simulink library "mahoneyAHRSlibrary"  (R2014a)
settings: Solver=ode45  StartTime=0.0  StopTime=10.0  RelTol=1e-3
values from neighbouring files (symbols this model uses):
  controlDT = 1 / 500    (= 0.002)    [setup.m]
undefined symbols (not defined in the file or in its folder): DiscIntNeverNeededParam
libraries: aerolibutil x8, simulink x3, mahoneyAHRSlibrary x1, aerolibtransform2 x1
settings Model: Creator=e722209  LastModifiedBy=John Ihlein

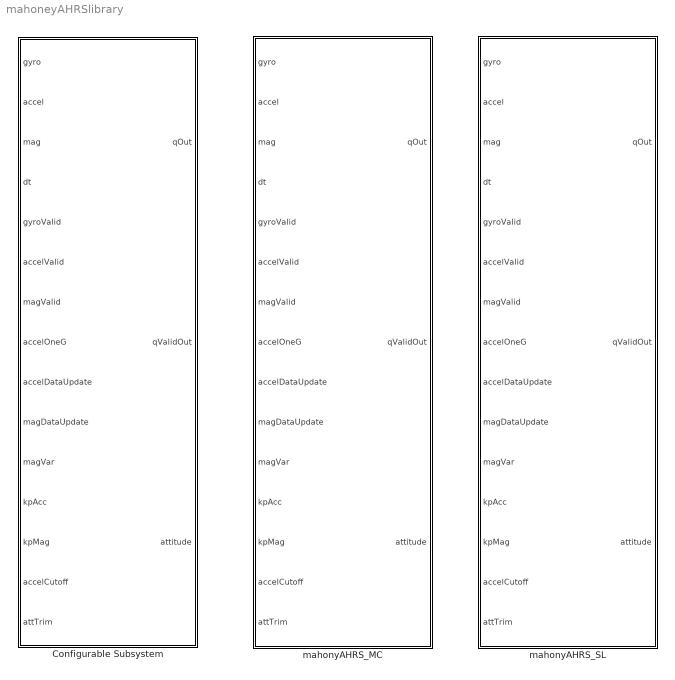
== system mahoneyAHRSlibrary ==
  Configurable Subsystem : Subsystem  BlockChoice=mahonyAHRS_MC
      settings: TemplateBlock=self  MemberBlocks=mahonyAHRS_MC,mahonyAHRS_SL
  mahonyAHRS_MC : MATLAB Function  TreatAsAtomicUnit=on
  mahonyAHRS_SL : Subsystem  TreatAsAtomicUnit=on

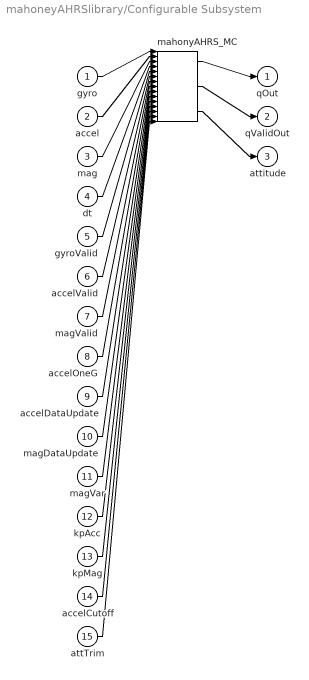
== system mahoneyAHRSlibrary/Configurable Subsystem ==
  gyro : Inport
  accel : Inport  Port=2
  mag : Inport  Port=3
  dt : Inport  Port=4
  gyroValid : Inport  Port=5
  accelValid : Inport  Port=6
  magValid : Inport  Port=7
  accelOneG : Inport  Port=8
  accelDataUpdate : Inport  Port=9
  magDataUpdate : Inport  Port=10
  magVar : Inport  Port=11
  kpAcc : Inport  Port=12
  kpMag : Inport  Port=13
  accelCutoff : Inport  Port=14
  attTrim : Inport  Port=15
  mahonyAHRS_MC : mahoneyAHRSlibrary/mahonyAHRS_MC
  qOut : Outport
  qValidOut : Outport  Port=2
  attitude : Outport  Port=3
  wires:
  gyro/1 -> mahonyAHRS_MC/1
  accel/1 -> mahonyAHRS_MC/2
  mag/1 -> mahonyAHRS_MC/3
  dt/1 -> mahonyAHRS_MC/4
  gyroValid/1 -> mahonyAHRS_MC/5
  accelValid/1 -> mahonyAHRS_MC/6
  magValid/1 -> mahonyAHRS_MC/7
  accelOneG/1 -> mahonyAHRS_MC/8
  accelDataUpdate/1 -> mahonyAHRS_MC/9
  magDataUpdate/1 -> mahonyAHRS_MC/10
  magVar/1 -> mahonyAHRS_MC/11
  kpAcc/1 -> mahonyAHRS_MC/12
  kpMag/1 -> mahonyAHRS_MC/13
  accelCutoff/1 -> mahonyAHRS_MC/14
  attTrim/1 -> mahonyAHRS_MC/15
  mahonyAHRS_MC/1 -> qOut/1
  mahonyAHRS_MC/2 -> qValidOut/1
  mahonyAHRS_MC/3 -> attitude/1

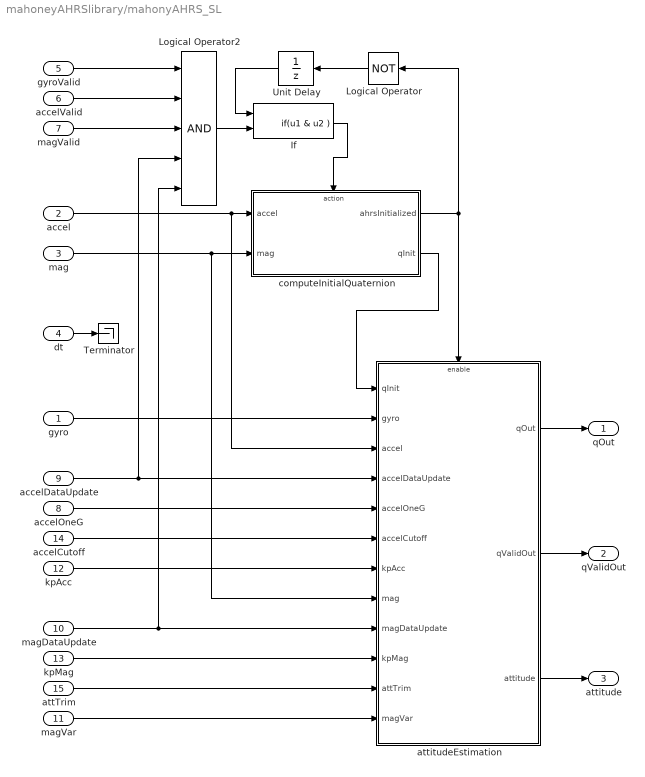
== system mahoneyAHRSlibrary/mahonyAHRS_SL ==
  gyro : Inport
  accel : Inport  Port=2
  mag : Inport  Port=3
  dt : Inport  Port=4
  gyroValid : Inport  Port=5
  accelValid : Inport  Port=6
  magValid : Inport  Port=7
  accelOneG : Inport  Port=8
  accelDataUpdate : Inport  Port=9
  magDataUpdate : Inport  Port=10
  magVar : Inport  Port=11
  kpAcc : Inport  Port=12
  kpMag : Inport  Port=13
  accelCutoff : Inport  Port=14
  attTrim : Inport  Port=15
  If : If  NumInputs=2  IfExpression=u1 & u2  ShowElse=off
  Logical Operator : Logic  Operator=NOT  IconShape=distinctive  AllPortsSameDT=off  OutDataTypeStr=boolean
  Logical Operator2 : Logic  Inputs=5  IconShape=distinctive  AllPortsSameDT=off  OutDataTypeStr=boolean
  Terminator : Terminator
  Unit Delay : UnitDelay  InitialCondition=1  SampleTime=-1
  attitudeEstimation : Subsystem  TreatAsAtomicUnit=on
  computeInitialQuaternion : Subsystem  TreatAsAtomicUnit=on
  qOut : Outport
  qValidOut : Outport  Port=2
  attitude : Outport  Port=3
  wires:
  magVar/1 -> attitudeEstimation/12(magVar)
  attTrim/1 -> attitudeEstimation/11(attTrim)
  attitudeEstimation/2(qValidOut) -> qValidOut/1
  attitudeEstimation/1(qOut) -> qOut/1
  Logical Operator/1 -> Unit Delay/1
  Logical Operator2/1 -> If/2
  computeInitialQuaternion/2(qInit) -> attitudeEstimation/1(qInit)
  Unit Delay/1 -> If/1
  computeInitialQuaternion/1(ahrsInitialized) -> Logical Operator/1, attitudeEstimation/Enable
  If/1 -> computeInitialQuaternion/Action
  attitudeEstimation/3(attitude) -> attitude/1
  accelDataUpdate/1 -> attitudeEstimation/4(accelDataUpdate), Logical Operator2/4
  magDataUpdate/1 -> attitudeEstimation/9(magDataUpdate), Logical Operator2/5
  accelOneG/1 -> attitudeEstimation/5(accelOneG)
  accelCutoff/1 -> attitudeEstimation/6(accelCutoff)
  accel/1 -> attitudeEstimation/3(accel), computeInitialQuaternion/1(accel)
  mag/1 -> attitudeEstimation/8(mag), computeInitialQuaternion/2(mag)
  gyro/1 -> attitudeEstimation/2(gyro)
  gyroValid/1 -> Logical Operator2/1
  magValid/1 -> Logical Operator2/3
  accelValid/1 -> Logical Operator2/2
  kpMag/1 -> attitudeEstimation/10(kpMag)
  kpAcc/1 -> attitudeEstimation/7(kpAcc)
  dt/1 -> Terminator/1

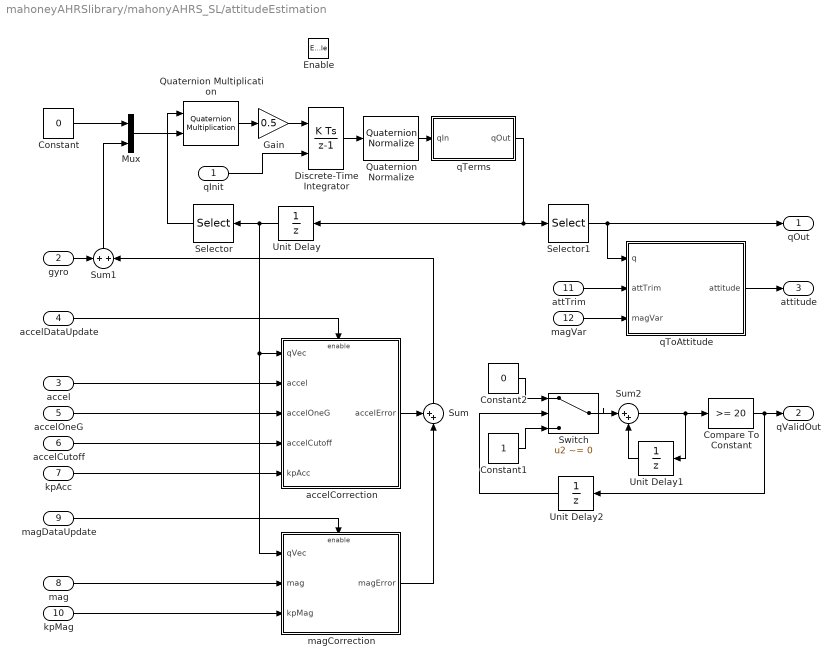
== system mahoneyAHRSlibrary/mahonyAHRS_SL/attitudeEstimation ==
  qInit : Inport
  gyro : Inport  Port=2
  accel : Inport  Port=3
  accelDataUpdate : Inport  Port=4
  accelOneG : Inport  Port=5
  accelCutoff : Inport  Port=6
  kpAcc : Inport  Port=7
  mag : Inport  Port=8
  magDataUpdate : Inport  Port=9
  kpMag : Inport  Port=10
  attTrim : Inport  Port=11
  magVar : Inport  Port=12
  Enable : EnablePort
  Compare To Constant : simulink/Logic and Bit Operations/Compare To Constant  relop=>=  const=20  OutDataTypeStr=uint8
  Constant : Constant  Value=0  OutDataTypeStr=single  SampleTime=controlDT
  Constant1 : Constant  OutDataTypeStr=single  SampleTime=controlDT
  Constant2 : Constant  Value=0  OutDataTypeStr=single  SampleTime=controlDT
  Discrete-Time Integrator : DiscreteIntegrator  InitialConditionSource=external  SampleTime=controlDT  ICPrevOutput=DiscIntNeverNeededParam  ICPrevScaledInput=DiscIntNeverNeededParam
  Gain : Gain  Gain=0.5
  Mux : Mux  Inputs=[1 3]
  Quaternion Multiplication : aerolibutil/Quaternion Multiplication
  Quaternion Normalize : aerolibutil/Quaternion Normalize
  Selector : Selector  InputPortWidth=14  Indices=[1:4]
  Selector1 : Selector  InputPortWidth=14  Indices=[1:4]
  Sum : Sum  Inputs=++|
  Sum1 : Sum  Inputs=+|+
  Sum2 : Sum  Inputs=|++
  Switch : Switch  Criteria=u2 ~= 0
  Unit Delay : UnitDelay  InitialCondition=[1 0 0 0 1 0 0 0 0 0 0 0 0 0]  SampleTime=-1
  Unit Delay1 : UnitDelay  SampleTime=-1
  Unit Delay2 : UnitDelay  SampleTime=-1
  accelCorrection : Subsystem  TreatAsAtomicUnit=on
  magCorrection : Subsystem  TreatAsAtomicUnit=on
  qTerms : Subsystem
  qToAttitude : Subsystem
  qOut : Outport  InitialOutput=[1 0 0 0]
  qValidOut : Outport  Port=2
  attitude : Outport  Port=3
  wires:
  magVar/1 -> qToAttitude/3(magVar)
  attTrim/1 -> qToAttitude/2(attTrim)
  qToAttitude/1(attitude) -> attitude/1
  Unit Delay2/1 -> Switch/2
  Compare To Constant/1 -> Unit Delay2/1, qValidOut/1
  Sum2/1 -> Unit Delay1/1, Compare To Constant/1
  Constant2/1 -> Switch/1
  Constant1/1 -> Switch/3
  Switch/1 -> Sum2/1
  Unit Delay1/1 -> Sum2/2
  Constant/1 -> Mux/1
  Mux/1 -> Quaternion Multiplication/2
  Unit Delay/1 -> accelCorrection/1(qVec), magCorrection/1(qVec), Selector/1
  Selector/1 -> Quaternion Multiplication/1
  Discrete-Time Integrator/1 -> Quaternion Normalize/1
  Selector1/1 -> qOut/1, qToAttitude/1(q)
  Quaternion Normalize/1 -> qTerms/1(qIn)
  qTerms/1(qOut) -> Selector1/1, Unit Delay/1
  qInit/1 -> Discrete-Time Integrator/2
  mag/1 -> magCorrection/2(mag)
  accel/1 -> accelCorrection/2(accel)
  accelOneG/1 -> accelCorrection/3(accelOneG)
  accelCutoff/1 -> accelCorrection/4(accelCutoff)
  Quaternion Multiplication/1 -> Gain/1
  Gain/1 -> Discrete-Time Integrator/1
  gyro/1 -> Sum1/1
  Sum1/1 -> Mux/2
  Sum/1 -> Sum1/2
  accelCorrection/1(accelError) -> Sum/1
  accelDataUpdate/1 -> accelCorrection/Enable
  magCorrection/1(magError) -> Sum/2
  magDataUpdate/1 -> magCorrection/Enable
  kpAcc/1 -> accelCorrection/5(kpAcc)
  kpMag/1 -> magCorrection/3(kpMag)

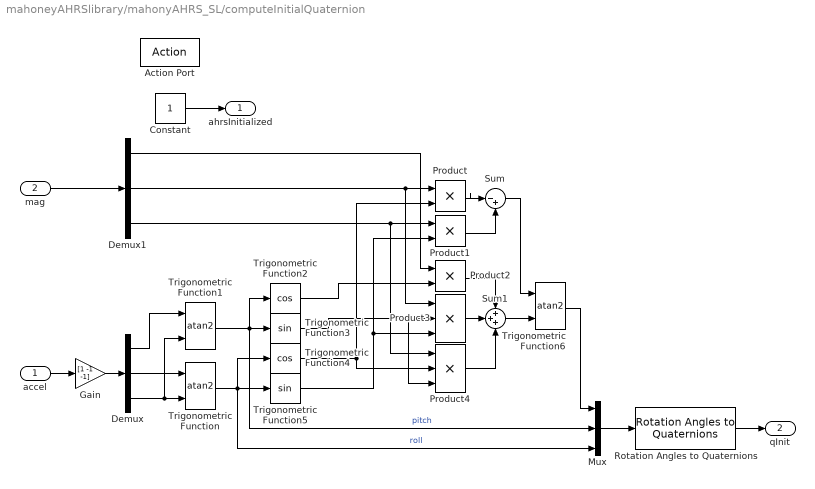
== system mahoneyAHRSlibrary/mahonyAHRS_SL/computeInitialQuaternion ==
  accel : Inport
  mag : Inport  Port=2
  Action Port : ActionPort
  Constant : Constant  OutDataTypeStr=uint8
  Demux : Demux  Outputs=3
  Demux1 : Demux  Outputs=3
  Gain : Gain  Gain=[1 -1 -1]
  Mux : Mux  Inputs=3
  Product : Product
  Product1 : Product
  Product2 : Product
  Product3 : Product  Inputs=3
  Product4 : Product  Inputs=3
  Rotation Angles to Quaternions : aerolibtransform2/Rotation Angles to Quaternions  rotationOrder=ZYX
  Sum : Sum  Inputs=|-+
  Sum1 : Sum  Inputs=+++
  Trigonometric Function : Trigonometry  Operator=atan2
  Trigonometric Function1 : Trigonometry  Operator=atan2
  Trigonometric Function2 : Trigonometry  Operator=cos
  Trigonometric Function3 : Trigonometry
  Trigonometric Function4 : Trigonometry  Operator=cos
  Trigonometric Function5 : Trigonometry
  Trigonometric Function6 : Trigonometry  Operator=atan2
  ahrsInitialized : Outport  InitialOutput=0
  qInit : Outport  Port=2  InitialOutput=[1 0 0 0]
  wires:
  Constant/1 -> ahrsInitialized/1
  accel/1 -> Gain/1
  Gain/1 -> Demux/1
  Demux/3 -> Trigonometric Function1/2, Trigonometric Function/2
  Demux/2 -> Trigonometric Function/1
  Demux/1 -> Trigonometric Function1/1
  Trigonometric Function/1 -> Mux/3, Trigonometric Function4/1, Trigonometric Function5/1  "roll"
  Trigonometric Function1/1 -> Trigonometric Function2/1, Mux/2, Trigonometric Function3/1  "pitch"
  mag/1 -> Demux1/1
  Demux1/2 -> Product3/1, Product/1
  Trigonometric Function4/1 -> Product4/2, Product/2
  Demux1/3 -> Product4/1, Product1/1
  Trigonometric Function5/1 -> Product3/3, Product1/2
  Product/1 -> Sum/1
  Product1/1 -> Sum/2
  Demux1/1 -> Product2/1
  Trigonometric Function2/1 -> Product2/2
  Trigonometric Function3/1 -> Product4/3, Product3/2
  Product3/1 -> Sum1/2
  Product2/1 -> Sum1/1
  Product4/1 -> Sum1/3
  Sum1/1 -> Trigonometric Function6/2
  Sum/1 -> Trigonometric Function6/1
  Mux/1 -> Rotation Angles to Quaternions/1
  Trigonometric Function6/1 -> Mux/1
  Rotation Angles to Quaternions/1 -> qInit/1

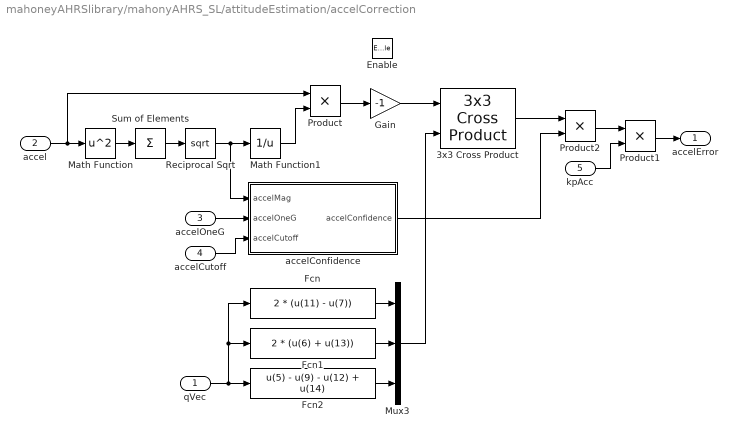
== system mahoneyAHRSlibrary/mahonyAHRS_SL/attitudeEstimation/accelCorrection ==
  qVec : Inport
  accel : Inport  Port=2
  accelOneG : Inport  Port=3
  accelCutoff : Inport  Port=4
  kpAcc : Inport  Port=5
  Enable : EnablePort
  3x3 Cross Product : aerolibutil/3x3 Cross Product
  Fcn : Fcn  Expr=2 * (u(11) - u(7))
  Fcn1 : Fcn  Expr=2 * (u(6) + u(13))
  Fcn2 : Fcn  Expr=u(5) - u(9) - u(12) + u(14)
  Gain : Gain  Gain=-1
  Math Function : Math  Operator=square  SaturateOnIntegerOverflow=on
  Math Function1 : Math  Operator=reciprocal  SaturateOnIntegerOverflow=on
  Mux3 : Mux  Inputs=3
  Product : Product
  Product1 : Product
  Product2 : Product
  Reciprocal Sqrt : Sqrt  SaturateOnIntegerOverflow=on
  Sum of Elements : Sum  Inputs=+
  accelConfidence : Subsystem
  accelError : Outport
  wires:
  accel/1 -> Product/1, Math Function/1
  Math Function/1 -> Sum of Elements/1
  Sum of Elements/1 -> Reciprocal Sqrt/1
  Reciprocal Sqrt/1 -> accelConfidence/1(accelMag), Math Function1/1
  Math Function1/1 -> Product/2
  accelOneG/1 -> accelConfidence/2(accelOneG)
  accelCutoff/1 -> accelConfidence/3(accelCutoff)
  Fcn/1 -> Mux3/1
  Fcn1/1 -> Mux3/2
  Fcn2/1 -> Mux3/3
  qVec/1 -> Fcn1/1, Fcn/1, Fcn2/1
  Product/1 -> Gain/1
  Gain/1 -> 3x3 Cross Product/1
  Mux3/1 -> 3x3 Cross Product/2
  Product2/1 -> Product1/1
  kpAcc/1 -> Product1/2
  Product1/1 -> accelError/1
  accelConfidence/1(accelConfidence) -> Product2/2
  3x3 Cross Product/1 -> Product2/1

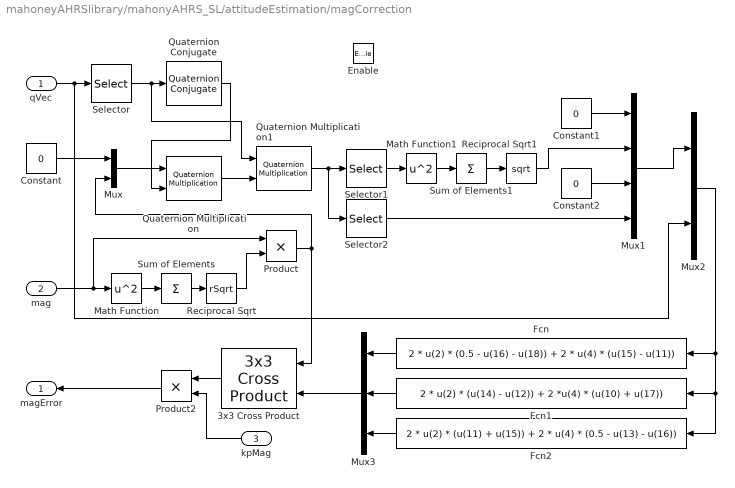
== system mahoneyAHRSlibrary/mahonyAHRS_SL/attitudeEstimation/magCorrection ==
  qVec : Inport
  mag : Inport  Port=2
  kpMag : Inport  Port=3
  Enable : EnablePort
  3x3 Cross Product : aerolibutil/3x3 Cross Product
  Constant : Constant  Value=0  OutDataTypeStr=single  SampleTime=controlDT
  Constant1 : Constant  Value=0  OutDataTypeStr=single  SampleTime=controlDT
  Constant2 : Constant  Value=0  OutDataTypeStr=single  SampleTime=controlDT
  Fcn : Fcn  Expr=2 * u(2) * (0.5 - u(16) - u(18)) + 2 * u(4) * (u(15) - u(11))
  Fcn1 : Fcn  Expr=2 * u(2) * (u(14) - u(12)) + 2 *u(4) * (u(10) + u(17))
  Fcn2 : Fcn  Expr=2 * u(2) * (u(11) + u(15)) + 2 * u(4) * (0.5 - u(13) - u(16))
  Math Function : Math  Operator=square  SaturateOnIntegerOverflow=on
  Math Function1 : Math  Operator=square  SaturateOnIntegerOverflow=on
  Mux : Mux  Inputs=[1 3]
  Mux1 : Mux
  Mux2 : Mux  Inputs=2
  Mux3 : Mux  Inputs=3
  Product : Product
  Product2 : Product
  Quaternion Conjugate : aerolibutil/Quaternion Conjugate
  Quaternion Multiplication : aerolibutil/Quaternion Multiplication
  Quaternion Multiplication1 : aerolibutil/Quaternion Multiplication
  Reciprocal Sqrt : Sqrt  Operator=rSqrt  SaturateOnIntegerOverflow=on
  Reciprocal Sqrt1 : Sqrt  SaturateOnIntegerOverflow=on
  Selector : Selector  InputPortWidth=14  Indices=[1:4]
  Selector1 : Selector  InputPortWidth=4  Indices=[2 3]
  Selector2 : Selector  InputPortWidth=4  Indices=4
  Sum of Elements : Sum  Inputs=+
  Sum of Elements1 : Sum  Inputs=+
  magError : Outport
  wires:
  qVec/1 -> Mux2/2, Selector/1
  mag/1 -> Product/1, Math Function/1
  Math Function/1 -> Sum of Elements/1
  Sum of Elements/1 -> Reciprocal Sqrt/1
  Reciprocal Sqrt/1 -> Product/2
  Constant/1 -> Mux/1
  Mux/1 -> Quaternion Multiplication/1
  Selector/1 -> Quaternion Multiplication1/1, Quaternion Conjugate/1
  Quaternion Conjugate/1 -> Quaternion Multiplication/2
  Quaternion Multiplication/1 -> Quaternion Multiplication1/2
  Selector1/1 -> Math Function1/1
  Math Function1/1 -> Sum of Elements1/1
  Sum of Elements1/1 -> Reciprocal Sqrt1/1
  Product/1 -> Mux/2, 3x3 Cross Product/1
  Quaternion Multiplication1/1 -> Selector2/1, Selector1/1
  Reciprocal Sqrt1/1 -> Mux1/2
  Constant2/1 -> Mux1/3
  Constant1/1 -> Mux1/1
  Selector2/1 -> Mux1/4
  Mux1/1 -> Mux2/1
  Mux2/1 -> Fcn2/1, Fcn1/1, Fcn/1
  Fcn/1 -> Mux3/1
  Fcn1/1 -> Mux3/2
  Fcn2/1 -> Mux3/3
  3x3 Cross Product/1 -> Product2/1
  Product2/1 -> magError/1
  Mux3/1 -> 3x3 Cross Product/2
  kpMag/1 -> Product2/2

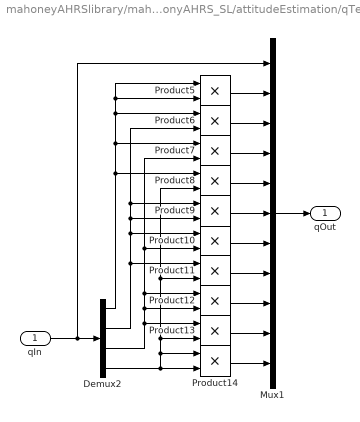
== system mahoneyAHRSlibrary/mahonyAHRS_SL/attitudeEstimation/qTerms ==
  qIn : Inport
  Demux2 : Demux
  Mux1 : Mux  Inputs=[4 1 1 1 1 1 1 1 1 1 1]
  Product{5..14} (10 alike) : Product
  qOut : Outport
  wires:
  Demux2/3 -> Product13/1, Product12/2, Product12/1, Product10/2, Product7/2
  Product7/1 -> Mux1/4
  Product10/1 -> Mux1/7
  Mux1/1 -> qOut/1
  Product11/1 -> Mux1/8
  Product6/1 -> Mux1/3
  Product5/1 -> Mux1/2
  Demux2/4 -> Product14/2, Product14/1, Product13/2, Product11/2, Product8/2
  Product14/1 -> Mux1/11
  Product12/1 -> Mux1/9
  qIn/1 -> Demux2/1, Mux1/1
  Product13/1 -> Mux1/10
  Product8/1 -> Mux1/5
  Product9/1 -> Mux1/6
  Demux2/1 -> Product8/1, Product7/1, Product6/1, Product5/2, Product5/1
  Demux2/2 -> Product11/1, Product10/1, Product9/2, Product9/1, Product6/2

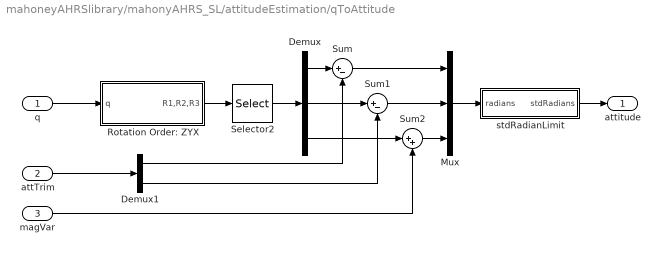
== system mahoneyAHRSlibrary/mahonyAHRS_SL/attitudeEstimation/qToAttitude ==
  q : Inport
  attTrim : Inport  Port=2
  magVar : Inport  Port=3
  Demux : Demux  Outputs=3
  Demux1 : Demux  Outputs=2
  Mux : Mux  Inputs=3
  Rotation Order: ZYX : Subsystem
  Selector2 : Selector  InputPortWidth=3  Indices=[3 2 1]
  Sum : Sum  Inputs=|+-
  Sum1 : Sum  Inputs=|+-
  Sum2 : Sum  Inputs=|++
  stdRadianLimit : Subsystem
  attitude : Outport
  wires:
  attTrim/1 -> Demux1/1
  magVar/1 -> Sum2/2
  Demux1/2 -> Sum1/2
  Demux1/1 -> Sum/2
  Demux/3 -> Sum2/1
  Sum1/1 -> Mux/2
  Demux/2 -> Sum1/1
  Demux/1 -> Sum/1
  Sum/1 -> Mux/1
  Sum2/1 -> Mux/3
  Selector2/1 -> Demux/1
  Mux/1 -> stdRadianLimit/1(radians)
  q/1 -> Rotation Order: ZYX/1(q)
  stdRadianLimit/1(stdRadians) -> attitude/1
  Rotation Order: ZYX/1(R1,R2,R3) -> Selector2/1

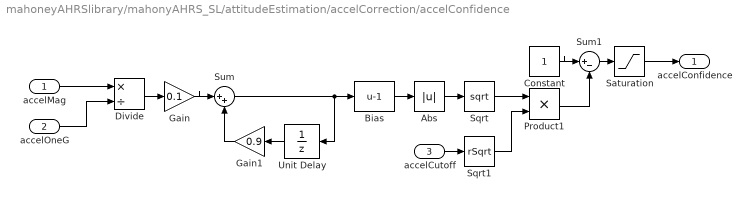
== system mahoneyAHRSlibrary/mahonyAHRS_SL/attitudeEstimation/accelCorrection/accelConfidence ==
  accelMag : Inport
  accelOneG : Inport  Port=2
  accelCutoff : Inport  Port=3
  Abs : Abs
  Bias : Bias  Bias=-1
  Constant : Constant  OutDataTypeStr=single  SampleTime=controlDT
  Divide : Product  Inputs=*/
  Gain : Gain  Gain=0.1
  Gain1 : Gain  Gain=0.9
  Product1 : Product
  Saturation : Saturate  UpperLimit=1  LowerLimit=0
  Sqrt : Sqrt  SaturateOnIntegerOverflow=on
  Sqrt1 : Sqrt  Operator=rSqrt  SaturateOnIntegerOverflow=on
  Sum : Sum  Inputs=|++
  Sum1 : Sum  Inputs=|+-
  Unit Delay : UnitDelay  InitialCondition=1  SampleTime=-1
  accelConfidence : Outport
  wires:
  Gain1/1 -> Sum/2
  Abs/1 -> Sqrt/1
  Gain/1 -> Sum/1
  Divide/1 -> Gain/1
  Bias/1 -> Abs/1
  Unit Delay/1 -> Gain1/1
  Sum/1 -> Bias/1, Unit Delay/1
  Product1/1 -> Sum1/2
  Sqrt/1 -> Product1/1
  accelCutoff/1 -> Sqrt1/1
  Constant/1 -> Sum1/1
  Sum1/1 -> Saturation/1
  accelOneG/1 -> Divide/2
  Saturation/1 -> accelConfidence/1
  accelMag/1 -> Divide/1
  Sqrt1/1 -> Product1/2

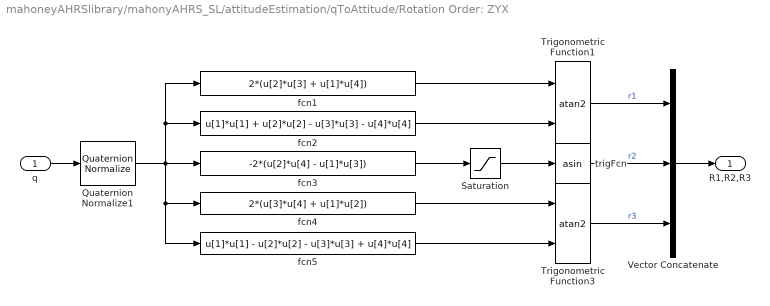
== system mahoneyAHRSlibrary/mahonyAHRS_SL/attitudeEstimation/qToAttitude/Rotation Order: ZYX ==
  q : Inport
  Quaternion Normalize1 : aerolibutil/Quaternion Normalize
  Saturation : Saturate  UpperLimit=1  LowerLimit=-1
  Trigonometric Function1 : Trigonometry  Operator=atan2
  Trigonometric Function3 : Trigonometry  Operator=atan2
  Vector Concatenate : Concatenate  NumInputs=3
  fcn1 : Fcn  Expr=2*(u[2]*u[3] + u[1]*u[4])
  fcn2 : Fcn  Expr=u[1]*u[1] + u[2]*u[2] - u[3]*u[3] - u[4]*u[4]
  fcn3 : Fcn  Expr=-2*(u[2]*u[4] - u[1]*u[3])
  fcn4 : Fcn  Expr=2*(u[3]*u[4] + u[1]*u[2])
  fcn5 : Fcn  Expr=u[1]*u[1] - u[2]*u[2] - u[3]*u[3] + u[4]*u[4]
  trigFcn : Trigonometry  Operator=asin
  R1,R2,R3 : Outport
  wires:
  Quaternion Normalize1/1 -> fcn3/1, fcn4/1, fcn5/1, fcn2/1, fcn1/1
  Trigonometric Function3/1 -> Vector Concatenate/3  "r3"
  trigFcn/1 -> Vector Concatenate/2  "r2"
  Trigonometric Function1/1 -> Vector Concatenate/1  "r1"
  Vector Concatenate/1 -> R1,R2,R3/1
  q/1 -> Quaternion Normalize1/1
  fcn3/1 -> Saturation/1
  fcn1/1 -> Trigonometric Function1/1
  fcn2/1 -> Trigonometric Function1/2
  fcn4/1 -> Trigonometric Function3/1
  fcn5/1 -> Trigonometric Function3/2
  Saturation/1 -> trigFcn/1

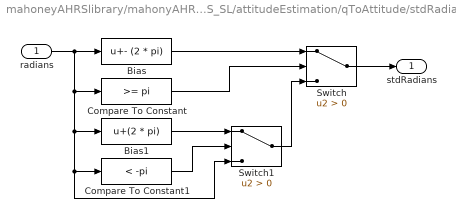
== system mahoneyAHRSlibrary/mahonyAHRS_SL/attitudeEstimation/qToAttitude/stdRadianLimit ==
  radians : Inport
  Bias : Bias  Bias=- (2 * pi)
  Bias1 : Bias  Bias=(2 * pi)
  Compare To Constant : simulink/Logic and Bit Operations/Compare To Constant  relop=>=  const=pi  OutDataTypeStr=boolean
  Compare To Constant1 : simulink/Logic and Bit Operations/Compare To Constant  relop=<  const=-pi  OutDataTypeStr=boolean
  Switch : Switch  Criteria=u2 > Threshold
  Switch1 : Switch  Criteria=u2 > Threshold
  stdRadians : Outport
  wires:
  Switch/1 -> stdRadians/1
  radians/1 -> Bias/1, Compare To Constant/1, Bias1/1, Compare To Constant1/1, Switch1/3
  Switch1/1 -> Switch/3
  Compare To Constant1/1 -> Switch1/2
  Bias1/1 -> Switch1/1
  Bias/1 -> Switch/1
  Compare To Constant/1 -> Switch/2

== matlab function mahoneyAHRSlibrary/mahonyAHRS_MC ==
  data: gyro input; qOut output; accel input; mag input; dt input; gyroValid input; accelValid input; magValid input; accelOneG input; accelDataUpdate input; magDataUpdate input; magVar input; kpAcc input; kpMag input; qValidOut output; accelCutoff input; attitude output; attTrim input
%%%%%%%%%%%%%%%%%%%%%%%%%%%%%%%%%%%%%%%%%%%%%%%%%%%%%%%%%%%%%%%%%%%%%%%
% MAYHONYAHRS Madgwick's implementation of Mayhony's AHRS algorithm
%
%   Date          Author          Notes
%   28/09/2011    SOH Madgwick    Initial release
%   25/08/2014    J Ihlein        Integrated into FF32
%%%%%%%%%%%%%%%%%%%%%%%%%%%%%%%%%%%%%%%%%%%%%%%%%%%%%%%%%%%%%%%%%%%%%%%

function [qOut, qValidOut, attitude] = mahonyAHRS(gyro, accel, mag, dt,...
                                                  gyroValid, accelValid, magValid,...
                                                  accelOneG, accelDataUpdate,...
                                                  magDataUpdate, magVar, ...
                                                  kpAcc, kpMag, accelCutoff, attTrim)
%#codegen

%%%%%%%%%%%%%%%%%%%%%%%%%%%%%%%%%%%%%%%%%%%%%%%%%%%%%%%%%%%

persistent accelConfidenceDecay ahrsFirstPass eAcc eMag pastAccelFilter
persistent q qValid qValidCount
persistent q1q1 q1q2 q1q3 q1q4 
persistent q2q2 q2q3 q2q4
persistent q3q3 q3q4
persistent q4q4

if isempty(ahrsFirstPass)
    accelConfidenceDecay = single(0);
    ahrsFirstPass        = uint8(1);
    eAcc                 = single([0 0 0]');
    eMag                 = single([0 0 0]');
    pastAccelFilter      = single(1);
    q                    = single([1 0 0 0]);
    qValid               = uint8(0);
    qValidCount          = uint8(0);
    
    q1q1 = single(1);
    q1q2 = single(0);
    q1q3 = single(0);
    q1q4 = single(0);
    q2q2 = single(0);
    q2q3 = single(0);
    q2q4 = single(0);
    q3q3 = single(0);
    q3q4 = single(0);
    q4q4 = single(0);
end

%%%%%%%%%%%%%%%%%%%%%%%%%%%%%%%%%%%%%%%%%%%%%%%%%%%%%%%%%%%

attitude = single([0 0 0]);

%%%%%%%%%%%%%%%%%%%%%%%%%%%%%%%%%%%%%%%%%%%%%%%%%%%%%%%%%%%

if ahrsFirstPass && accelValid && accelDataUpdate && gyroValid && magValid && magDataUpdate
    initialRoll  = atan2(-accel(2), -accel(3));
    initialPitch = atan2( accel(1), -accel(3));
    
    cosRoll  = cos(initialRoll);
    sinRoll  = sin(initialRoll);
    cosPitch = cos(initialPitch);
    sinPitch = sin(initialPitch);
    
    magX = mag(1) * cosPitch + mag(2) * sinRoll * sinPitch + mag(3) * cosRoll * sinPitch;
    magY = mag(2) * cosRoll - mag(3) * sinRoll;
    
    initialHdg = atan2(-magY, magX);
    
    u1 = sin(initialHdg   / 2);
    u2 = sin(initialPitch / 2);
    u3 = sin(initialRoll  / 2);
    u4 = cos(initialHdg   / 2);
    u5 = cos(initialPitch / 2);
    u6 = cos(initialRoll  / 2);
    
    q(1) = u4 * u5 * u6 + u1 * u2 * u3;
    q(2) = u4 * u5 * u3 - u1 * u2 * u6;
    q(3) = u4 * u2 * u6 + u1 * u5 * u3;
    q(4) = u1 * u5 * u6 - u4 * u2 * u3;
    
    q1q1 = q(1) * q(1);
    q1q2 = q(1) * q(2);
    q1q3 = q(1) * q(3);
    q1q4 = q(1) * q(4);
    q2q2 = q(2) * q(2);
    q2q3 = q(2) * q(3);
    q2q4 = q(2) * q(4);
    q3q3 = q(3) * q(3);
    q3q4 = q(3) * q(4);
    q4q4 = q(4) * q(4);
    
    accelConfidenceDecay = single(1) / sqrt(accelCutoff);
    
    ahrsFirstPass = uint8(0);
end

%%%%%%%%%%%%%%%%%%%%%%%%%%%%%%%%%%%%%%%%%%%%%%%%%%%%%%%%%%%

if ~ahrsFirstPass
    if accelDataUpdate
        %Normalise accelerometer measurement
        accelNorm = norm(accel);
        % if(accelNorm == 0), return; end   % handle NaN
        accel = accel / accelNorm;          % normalise magnitude
        
        input = accelNorm / accelOneG;
        output = 0.1 * input + 0.9 * pastAccelFilter;
        pastAccelFilter = output;
        accelConfidence = 1 - (accelConfidenceDecay * sqrt(abs(output - 1)));
        
        if accelConfidence > 1
            accelConfidence = single(1);
        elseif accelConfidence < 0
            accelConfidence = single(0);
        end
        
        % Estimated direction of gravity and magnetic field
        v = [2 * (q2q4 - q1q3)
             2 * (q1q2 + q3q4)
             q1q1 - q2q2 - q3q3 + q4q4];
        
        % Error is sum of cross product between estimated direction and measured direction of fields
        eAcc = cross(-accel, v) * kpAcc * accelConfidence;
    end
    
    %%%%%%%%%%%%%%%%%%%%%%%%%%%%%%%%%%%%%%%%%%%%%%%%%%%%%%%
    
    if magDataUpdate
        % Normalise magnetometer measurement
        % if(norm(mag) == 0), return; end     % handle NaN
        mag = mag / norm(mag);                % normalise magnitude
        
        % Reference direction of Earth's magnetic field
        h = quaternProd(q, quaternProd([0 mag'], quaternConj(q)));
        b = [0 norm([h(2) h(3)]) 0 h(4)];
        
        w = [2 * b(2) * (0.5 - q3q3 - q4q4) + 2 * b(4) * (q2q4 - q1q3)
             2 * b(2) * (q2q3 - q1q4) + 2 * b(4) * (q1q2 + q3q4)
             2 * b(2) * (q1q3 + q2q4) + 2 * b(4) * (0.5 - q2q2 - q3q3)];
        
        % Error is sum of cross product between estimated direction and measured direction of fields
        eMag = cross(mag, w) * kpMag;
    end
    
    %%%%%%%%%%%%%%%%%%%%%%%%%%%%%%%%%%%%%%%%%%%%%%%%%%%%%%%
    
    % Apply feedback terms
    gyro = gyro + eAcc + eMag;
    
    % Compute rate of change of quaternion
    qDot = 0.5 * quaternProd(q, [0 gyro(1) gyro(2) gyro(3)]);
    
    % Integrate to yield quaternion
    q = q + qDot * dt;
    q = q / norm(q);
    
    qOut = q;
    
    if (qValid == 0)
        qValidCount = qValidCount + 1;
    end
    
    if ((qValidCount >= 20) && (qValid == 0))
        qValid = uint8(1);
    end
    
    qValidOut = qValid;
    
    q1q1 = q(1) * q(1);
    q1q2 = q(1) * q(2);
    q1q3 = q(1) * q(3);
    q1q4 = q(1) * q(4);
    q2q2 = q(2) * q(2);
    q2q3 = q(2) * q(3);
    q2q4 = q(2) * q(4);
    q3q3 = q(3) * q(3);
    q3q4 = q(3) * q(4);
    q4q4 = q(4) * q(4);
    
    %%%%%%%%%%%%%%%%%%%%%%%%%%%%%%%%%%%%%%%%%%%%%%%%%%%%%%%
    
    attitude(3) = atan2(2 * (q2q3 + q1q4), q1q1 + q2q2 - q3q3 - q4q4) + magVar;
    
    asinPitch = -2 * (q2q4 - q1q3);
    
    if asinPitch > 1
        asinPitch = single(1);
    elseif asinPitch < -1;
        asinPitch = single(-1);
    end
    
    attitude(2) = asin(asinPitch) - attTrim(2);
    
    attitude(1) = atan2(2 * (q3q4 + q1q2), q1q1 - q2q2 - q3q3 + q4q4) - attTrim(1);
    
    %%%%%%%%%%%%%%%%%%%%%%%%%%%%%%%%%%%%%%%%%%%%%%%%%%%%%%%
    
    if attitude(1) >= pi
        attitude(1) = attitude(1) - 2 * pi;
    elseif attitude(1) < -pi
        attitude(1) = attitude(1) + 2 * pi;
    end
    
    if attitude(2) >= pi
        attitude(2) = attitude(2) - 2 * pi;
    elseif attitude(2) < -pi
        attitude(2) = attitude(2) + 2 * pi;
        end
    
    if attitude(3) >= pi
        attitude(3) = attitude(3) - 2 * pi;
    elseif attitude(3) < -pi
        attitude(3) = attitude(3) + 2 * pi;
    end
    
    %%%%%%%%%%%%%%%%%%%%%%%%%%%%%%%%%%%%%%%%%%%%%%%%%%%%%%%
else
    qOut = single([1 0 0 0]);    
        
    qValidOut = uint8(0);
    
    q1q1 = single(1);
    q1q2 = single(0);
    q1q3 = single(0);
    q1q4 = single(0);
    q2q2 = single(0);
    q2q3 = single(0);
    q2q4 = single(0);
    q3q3 = single(0);
    q3q4 = single(0);
    q4q4 = single(0);   
    
    attitude(3) = 0;
    attitude(2) = 0;
    attitude(1) = 0;
end

end

%%%%%%%%%%%%%%%%%%%%%%%%%%%%%%%%%%%%%%%%%%%%%%%%%%%%%%%%%%%%%%%%%%%%%%%
%QUATERNCONJ Converts a quaternion to its conjugate
%
%   qConj = quaternConj(q)
%
%   Converts a quaternion to its conjugate.
%
%   Date          Author          Notes
%	27/09/2011    SOH Madgwick    Initial release
%   25/08/2014    J Ihlein        Integrated into FF32
%%%%%%%%%%%%%%%%%%%%%%%%%%%%%%%%%%%%%%%%%%%%%%%%%%%%%%%%%%%%%%%%%%%%%%%

function qConj = quaternConj(q)
%#codegen
    qConj = [q(1) -q(2) -q(3) -q(4)];
end

%%%%%%%%%%%%%%%%%%%%%%%%%%%%%%%%%%%%%%%%%%%%%%%%%%%%%%%%%%%%%%%%%%%%%%%
%QUATERNPROD Calculates the quaternion product
%
%   ab = quaternProd(a, b)
%
%   Calculates the quaternion product of quaternion a and b.
%
%   Date          Author          Notes
%	27/09/2011    SOH Madgwick    Initial release
%   25/08/2014    J Ihlein        Integrated into FF32
%%%%%%%%%%%%%%%%%%%%%%%%%%%%%%%%%%%%%%%%%%%%%%%%%%%%%%%%%%%%%%%%%%%%%%%

function ab = quaternProd(a, b)
%#codegen
    ab = zeros(1,4);
    
    ab(1) = a(1) * b(1) - a(2) * b(2) - a(3) * b(3) - a(4) * b(4);
    ab(2) = a(1) * b(2) + a(2) * b(1) + a(3) * b(4) - a(4) * b(3);
    ab(3) = a(1) * b(3) - a(2) * b(4) + a(3) * b(1) + a(4) * b(2);
    ab(4) = a(1) * b(4) + a(2) * b(3) - a(3) * b(2) + a(4) * b(1);
end

%%%%%%%%%%%%%%%%%%%%%%%%%%%%%%%%%%%%%%%%%%%%%%%%%%%%%%%%%%%%%%%%%%%%%%%
